simulink model "MCK"  (R2016b)
settings: Solver=VariableStepAuto  StartTime=0.0  StopTime=100  RelTol=1e-3
settings Model: Creator=Mojtaba  LastModifiedBy=Mojtaba

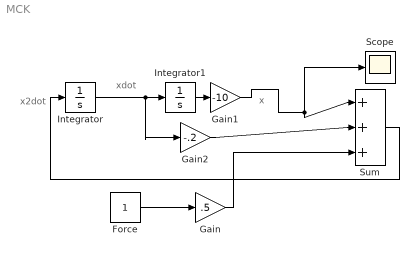
== system MCK ==
  note: x2dot
  note: x
  note: xdot
  Force : Constant
  Gain : Gain  Gain=.5
  Gain1 : Gain  Gain=-10
  Gain2 : Gain  Gain=-.2
  Integrator : Integrator
  Integrator1 : Integrator
  Scope : Scope
  Sum : Sum  Inputs=|+++
  wires:
  Integrator/1 -> Gain2/1, Integrator1/1
  Sum/1 -> Integrator/1
  Force/1 -> Gain/1
  Gain/1 -> Sum/3
  Integrator1/1 -> Gain1/1
  Gain1/1 -> Scope/1, Sum/1
  Gain2/1 -> Sum/2
